simulink model "Simulink_maniobra_2019a"  (R2020b)
settings: Solver=ode4  StartTime=0.0  StopTime=50000  FixedStep=0.05  RelTol=1e-100
values from neighbouring files (symbols this model uses):
  N_dr_H2N_0 = Euler3132C(angles_313_spacecraft)'*[0;vel_0_launch;0]    [Matlab_parametros.m]
  N_r_H2N_0 = Euler3132C(angles_313_spacecraft)'*[perigee_0;0;0]    [Matlab_parametros.m]
settings Model: SimulationMode=accelerator  Creator=Franklin  LastModifiedBy=Franklin
settings DebuggingCC: SFMachineParentedDataDiag=error

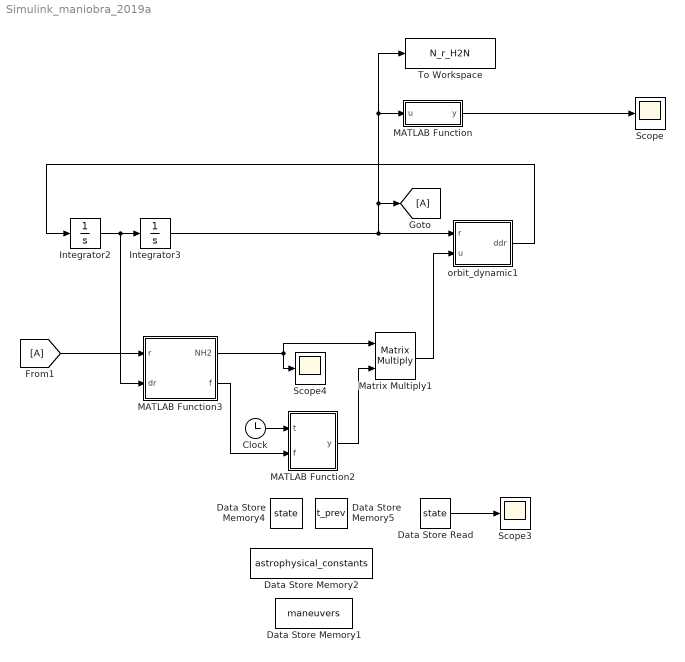
== system Simulink_maniobra_2019a ==
  Clock : Clock
  Data Store Memory1 : DataStoreMemory  DataStoreName=maneuvers  ReadBeforeWriteMsg=warning  WriteAfterWriteMsg=warning  WriteAfterReadMsg=warning  InitialValue=maneuvers  ShowAdditionalParam=off  OutDataTypeStr=double
  Data Store Memory2 : DataStoreMemory  DataStoreName=astrophysical_constants  ReadBeforeWriteMsg=warning  WriteAfterWriteMsg=warning  WriteAfterReadMsg=warning  InitialValue=astrophysical_constants  ShowAdditionalParam=off  OutDataTypeStr=double
  Data Store Memory4 : DataStoreMemory  DataStoreName=state  ReadBeforeWriteMsg=warning  WriteAfterWriteMsg=warning  WriteAfterReadMsg=warning  InitialValue=state  ShowAdditionalParam=off  OutDataTypeStr=int8
  Data Store Memory5 : DataStoreMemory  DataStoreName=t_prev  ReadBeforeWriteMsg=warning  WriteAfterWriteMsg=warning  WriteAfterReadMsg=warning  InitialValue=t_prev  ShowAdditionalParam=off  OutDataTypeStr=double
  Data Store Read : DataStoreRead  DataStoreName=state
  Integrator2 : Integrator  InitialCondition=N_dr_H2N_0
  Integrator3 : Integrator  InitialCondition=N_r_H2N_0
  MATLAB Function : MATLAB Function  TreatAsAtomicUnit=on
  MATLAB Function2 : MATLAB Function  TreatAsAtomicUnit=on
  MATLAB Function3 : MATLAB Function  TreatAsAtomicUnit=on
  Matrix Multiply1 : Product  Multiplication=Matrix(*)
  Scope : Scope
  Scope3 : Scope
  Scope4 : Scope
  To Workspace : ToWorkspace  VariableName=N_r_H2N  SampleTime=10
  orbit_dynamic1 : MATLAB Function  TreatAsAtomicUnit=on
  wires:
  Integrator2/1 -> MATLAB Function3/2(dr), Integrator3/1
  Integrator3/1 -> To Workspace/1, MATLAB Function/1(u), [A], orbit_dynamic1/1(r)
  orbit_dynamic1/1(ddr) -> Integrator2/1
  Clock/1 -> MATLAB Function2/1(t)
  [A] -> MATLAB Function3/1(r)
  MATLAB Function3/1(NH2) -> Scope4/1, Matrix Multiply1/1
  MATLAB Function/1(y) -> Scope/1
  Matrix Multiply1/1 -> orbit_dynamic1/2(u)
  MATLAB Function2/1(y) -> Matrix Multiply1/2
  MATLAB Function3/2(f) -> MATLAB Function2/2(f)
  Data Store Read/1 -> Scope3/1

== matlab function Simulink_maniobra_2019a/MATLAB Function ==
  data: u input; y output
function y = fcn(u)
y = norm(u);

== matlab function Simulink_maniobra_2019a/orbit_dynamic1 ==
  settings: updateMethod=DISCRETE
  data: r input; ddr output; astrophysical_constants data_store_memory; u input
function ddr = fcn(r,u)
global astrophysical_constants;

mu=astrophysical_constants(1,1);

ddr = -(mu/(norm(r)^3))*r+u;

== matlab function Simulink_maniobra_2019a/MATLAB Function2 ==
  settings: updateMethod=DISCRETE
  data: t input; f input; y output; astrophysical_constants data_store_memory; state data_store_memory; t_prev data_store_memory; maneuvers data_store_memory
function y = fcn(t,f)

global astrophysical_constants;
global state;
global t_prev;
global maneuvers;

y=zeros(3,1);
epsilon_f=0.0001;
dT=1;
if state==0 && t>=2000
    state=int8(1);
    t_prev=t;
    astrophysical_constants(5)=10;
end

if state==1
    if abs(f-0)<epsilon_f
        state=int8(2);
        t_prev=t;
    end
end

if state==2
    if t>=t_prev && t<t_prev+dT 
        dVA=maneuvers(1,1);
        y = [0;dVA/dT;0];
    end
    if t>t_prev+dT
        state=int8(3);
    end
end

if state==3
    if abs(f-pi)<epsilon_f
        state=int8(4);
        t_prev=t;
    end
end

if state==4
    if t>=t_prev && t<t_prev+dT
        dVB=maneuvers(2,1);
        y = [0;dVB/dT;0];
    end
    if t>t_prev+dT
        state=int8(5);
    end
end

if state==5
    if abs(f)<epsilon_f
        state=int8(6);
        t_prev=t;
    end
end

if state==6
    dT=1;
    if t>=t_prev && t<t_prev+dT 
        dVC=maneuvers(3,1);
        y = [0;dVC/dT;0];
    end
    if t>t_prev+dT
        state=int8(7);
    end
end

== matlab function Simulink_maniobra_2019a/MATLAB Function3 ==
  settings: updateMethod=DISCRETE
  data: r input; NH2 output; dr input; astrophysical_constants data_store_memory; f output
function [NH2,f] = fcn(r,dr)
global astrophysical_constants;
mu=astrophysical_constants(1,1);
a=astrophysical_constants(3,1); %apogee
b=astrophysical_constants(4,1); %perigee
e=(1-(b/a)^2)^0.5; %eccentricity
h_vector=cross(r,dr); %angular momentum
p=norm(h_vector)^2/mu;
c=cross(dr,h_vector)-mu*(r/norm(r)); %eccentricity vector momentum
f=acos(r'*c/(norm(r)*norm(c)));
if r'*dr<0
f=2*pi-f;
end
H2H1=eye(3);
H2H1(1:2,1:2)=(1/(1+e^2+2*e*cos(f))^0.5)*[1+e*cos(f),-e*sin(f);e*sin(f),1+e*cos(f)];

ir=r/norm(r);
ih=(cross(r,dr))/norm(cross(r,dr));
ith=cross(ih,ir);
H1N=[ir';ith';ih'];
NH2=H1N'*H2H1';
